simulink model "control_scheme"  (R2023b)
settings: Solver=VariableStepAuto  StartTime=0.0  StopTime=10.0  RelTol=1e-3
libraries: instrumentlib x2
settings Model: Creator=pc  LastModifiedBy=pc

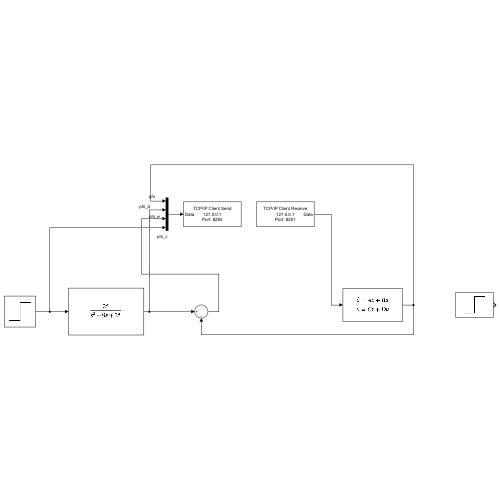
[thumbnail: Simulink's stored preview of the top-level diagram]
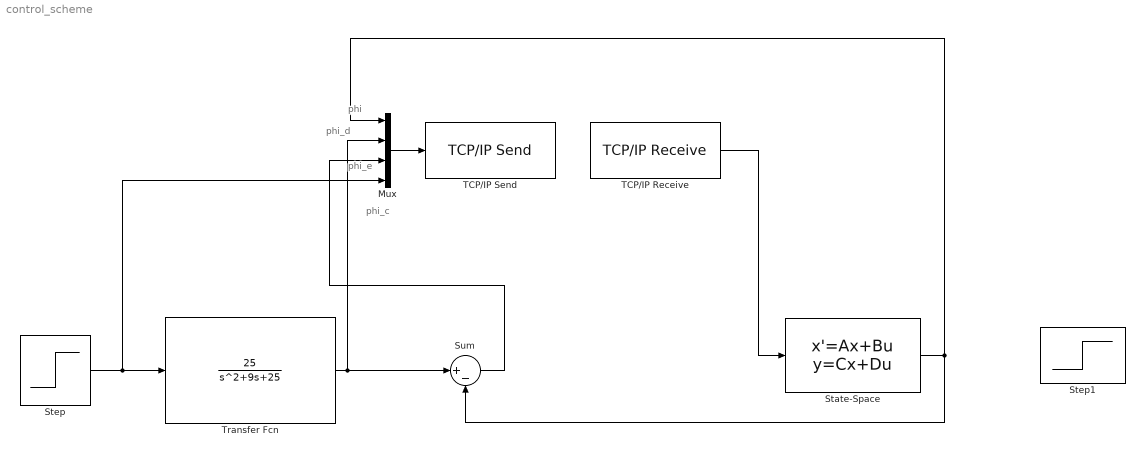
== system control_scheme ==
  note: phi
  note: phi_d
  note: phi_e
  note: phi_c
  Mux : Mux
  State-Space : StateSpace  InitialCondition=0  ContinuousStateAttributes='Controlled_Object'
  Step : Step  SampleTime=0
  Step1 : Step  SampleTime=0
  Sum : Sum  Inputs=|+-
  TCP/IP Receive : instrumentlib/TCP//IP Receive  Host=127.0.0.1  Port=8281  DataSize=[ 1 ]  DataType=double  ASCIIFormatting=%f  Terminator=LF  CustomTerminator=10  ByteOrder=big-endian  EnableBlockingMode=on  Timeout=10  SampleTime=0.01  SimulateUsing=Interpreted execution
  TCP/IP Send : instrumentlib/TCP//IP Send  Host=127.0.0.1  Port=8280  ByteOrder=big-endian  EnableBlockingMode=on  Timeout=10  TransferDelay=on  SimulateUsing=Interpreted execution
  Transfer Fcn : TransferFcn  Numerator=[25]  Denominator=[1 9 25]  ContinuousStateAttributes='Reference_Model'
  wires:
  Step/1 -> Mux/4, Transfer Fcn/1
  TCP/IP Receive/1 -> State-Space/1
  State-Space/1 -> Sum/2, Mux/1
  Mux/1 -> TCP/IP Send/1
  Transfer Fcn/1 -> Sum/1, Mux/2
  Sum/1 -> Mux/3
